simulink model "Pilote_SimMechanics"  (R2013a)
settings: Solver=ode15s  StartTime=0.0  StopTime=10.0  RelTol=1e-3
undefined symbols (not defined in the file): _EF_BancPH_ivan, RootGround, RootPart, SE_Bati, SE_Cylindre, SE_Safran
libraries: mblibv1 x14
settings Model: Creator=Ivan  LastModifiedBy=Ivan
settings SimMechanicsCC: VisOnUpdateDiagram=on  VisDuringSimulation=on

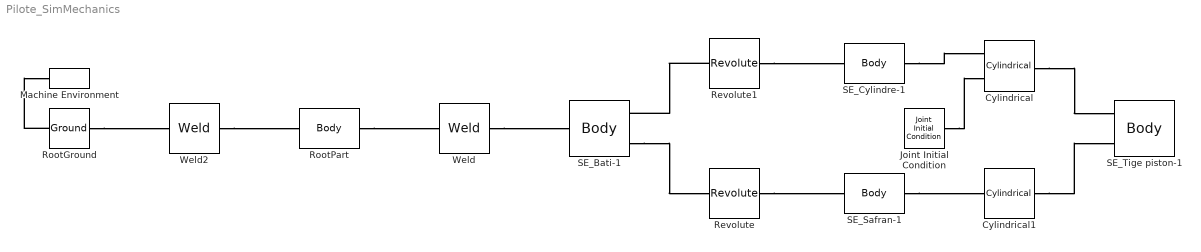
== system Pilote_SimMechanics ==
  Cylindrical : mblibv1/Joints/Cylindrical  LConnTagsString=__newl0|SA1  RConnTagsString=__newr0  UpdateFromCAD=on  PMImportedID=SE_Cylindre-1:-:SE_Tige piston-1  NumSAPorts=1  CutJoint=off  MarkAsCut=off  Primitives=prismatic  PrimitiveProps=P1$World$[-0.999105,-0.0423027,0]$prismatic#R1$World$[-0.999105,-0.0423027,0]$revolute  DialogClass=JointBlock  P1Axis=[-0.999105,-0.0423027,0]  R1Axis=[-0.999105,-0.0423027,0]
  Cylindrical1 : mblibv1/Joints/Cylindrical  LConnTagsString=__newl0  RConnTagsString=__newr0  UpdateFromCAD=on  PMImportedID=SE_Safran-1:-:SE_Tige piston-1  NumSAPorts=0  CutJoint=off  MarkAsCut=off  Primitives=prismatic  PrimitiveProps=P1$WORLD$[0,0,-1]$prismatic#R1$WORLD$[0,0,-1]$revolute  DialogClass=JointBlock  P1Axis=[0,0,-1]  R1Axis=[0,0,-1]
  Joint Initial Condition : mblibv1/Sensors &  Actuators/Joint Initial Condition  UpdateFromCAD=off  LeftPortType=blob  RightPortType=blob  PhysicalDomain=mechanical  DialogClass=InitialConditionBlock  InitialConditions=P1$true$0$m$deg$1$cm/s$deg/s#P2$false$0$m$deg$0$m/s$deg/s#P3$false$0$m$deg$0$m/s$deg/s#R1$false$0$m$deg$0$m/s$deg/s#R2$false$0$m$deg$0$m/s$deg/s#R3$false$0$m$deg$0$m/s$deg/s#S$false$0$m$deg$0$m/s$deg/s  P1PIC=0  P1VIC=1  P2PIC=0  P2VIC=0  P3PIC=0  P3VIC=0  R1PIC=0  R1VIC=0  R2PIC=0  R2VIC=0  R3PIC=0  R3VIC=0  SPIC=0  SVIC=0
  Machine Environment : mblibv1/Bodies/Machine Environment  PortType=env  PhysicalDomain=Mechanical  DialogTemplateClass=MECH.MachineEnvironment  SyncWhenCopied=off  Gravity=[0 0 -9.81]  GravityUnits=m/s^2  GravityAsSignal=off  Dimensionality=Auto-detect  AnalysisType=Forward dynamics  LinearAssemblyTolerance=1e-3  LinearAssemblyToleranceUnits=m  AngularAssemblyTolerance=1e-3  AngularAssemblyToleranceUnits=rad  ConstraintSolverType=Stabilizing  ConstraintRelTolerance=1e-4  ConstraintAbsTolerance=1e-4  UseRobustSingularityHandling=off  RedundancyAnalysisToleranceType=Automatically select tolerance  RedundancyAnalysisTolerance=1e-14  StatePerturbationType=Fixed  PerturbationSize=1e-5  VisualizeMachine=on  BodyVisualizationType=Use model default body geometries  BodyColorSelMode=Use model default  DefaultBodyColor=[1 0 0]
  Revolute : mblibv1/Joints/Revolute  LConnTagsString=__newl0  RConnTagsString=__newr0  UpdateFromCAD=on  PMImportedID=SE_Bati-1:-:SE_Safran-1  NumSAPorts=0  CutJoint=off  MarkAsCut=off  Primitives=prismatic  PrimitiveProps=R1$WORLD$[0,0,1]$revolute  DialogClass=JointBlock  R1Axis=[0,0,1]
  Revolute1 : mblibv1/Joints/Revolute  LConnTagsString=__newl0  RConnTagsString=__newr0  UpdateFromCAD=off  NumSAPorts=0  CutJoint=off  MarkAsCut=off  Primitives=prismatic  PrimitiveProps=R1$World$[0 0 1]$revolute  DialogClass=JointBlock  R1Axis=[0 0 1]
  RootGround : mblibv1/Bodies/Ground  UpdateFromCAD=on  PMImportedID=RootGround  LeftPortType=env  RightPortType=workingframe  PhysicalDomain=Mechanical  DialogClass=GroundBlock  CoordPosition=[-1.08828,0.614921,0.309081]  CoordPositionUnits=m  StateVectorMgrId=0  MachineId=[1 0]  ShowEnvPort=on
  RootPart : mblibv1/Bodies/Body  LConnTagsString=CS3  RConnTagsString=CS2  UpdateFromCAD=on  PMImportedID=_EF_BancPH_ivan/RootPart  DialogClass=MechanicalBodyBlock  Mass=0  MassUnits=kg  InertiaUnits=kg*m^2  Inertia=[0,0,0;0,0,0;0,0,0]  Shape=Cylinder  ShapeDims=[1 1]  ShapeUnits=m  ShapeUse=false  Density=1  DensityUnits=kg/m^3  DensityUse=false  GraphicsMode=MACHINE_DEFAULT  BodyColorSelMode=MACHINE_DEFAULT  BodyColor=[1;0;0]  AttachedToCS=CS1  CG=Right$CG$[-1.08828 0.614921 0.309081]$WORLD$WORLD$m$[1 0 0;0 1 0;0 0 1]$3x3 Transform$rad$WORLD$false$_EF_BancPH_ivan/RootPart::CG(AUTOGEN)  WorkingFrames=Right$CS1$[0 0 0]$WORLD$WORLD$m$[1 0 0;0 1 0;0 0 1]$3x3 Transform$rad$WORLD$false$_EF_BancPH_ivan/RootPart::CS1(AUTOGEN)#Right$CS2$[-1.08627 0.612468 0.301696]$WORLD$WORLD$m$[1 0 0;0 1 0;0 0 1]$3x3 Transform$rad$WORLD$true$SE_Bati-1:-:_EF_BancPH_ivan/RootPart::_EF_BancPH_ivan/RootPart(AUTOGEN)#Left$CS3$[-1.08828 0.614921 0.309081]$WORLD$WORLD$m$[1 0 0;0 1 0;0 0 1]$3x3 Transform$rad$WORLD$true$RootGround:-:_EF_BancPH_ivan/RootPart::_EF_BancPH_ivan/RootPart(AUTOGEN)  CGPos=[-1.08828 0.614921 0.309081]  CGRot=[1 0 0;0 1 0;0 0 1]  CS0Pos=[]  CS0Rot=[]  CS1Pos=[0 0 0]  CS1Rot=[1 0 0;0 1 0;0 0 1]  CS2Pos=[-1.08627 0.612468 0.301696]  CS2Rot=[1 0 0;0 1 0;0 0 1]  CS3Pos=[-1.08828 0.614921 0.309081]  CS3Rot=[1 0 0;0 1 0;0 0 1]  CS4Pos=[]  CS4Rot=[]  CS5Pos=[]  CS5Rot=[]  CS6Pos=[]  CS6Rot=[]  CS7Pos=[]  CS7Rot=[]  CS8Pos=[]  CS8Rot=[]  CS9Pos=[]  CS9Rot=[]  CS10Pos=[]  CS10Rot=[]  CS11Pos=[]  CS11Rot=[]  CS12Pos=[]  CS12Rot=[]  CS13Pos=[]  CS13Rot=[]  CS14Pos=[]  CS14Rot=[]  CS15Pos=[]  CS15Rot=[]  CS16Pos=[]  CS16Rot=[]  CS17Pos=[]  CS17Rot=[]  CS18Pos=[]  CS18Rot=[]  CS19Pos=[]  CS19Rot=[]  CS20Pos=[]  CS20Rot=[]
  SE_Bati-1 : mblibv1/Bodies/Body  LConnTagsString=CS2  RConnTagsString=CS3|CS4  UpdateFromCAD=on  PMImportedID=SE_Bati-1  DialogClass=MechanicalBodyBlock  Mass=10.7703  MassUnits=kg  InertiaUnits=kg*m^2  Inertia=[0.196607,0.0119133,0.0109935;0.0119133,1.14271,-0.000206125;0.0109935,-0.000206125,1.29701]  Shape=Cylinder  ShapeDims=[1 1]  ShapeUnits=m  ShapeUse=false  Density=1  DensityUnits=kg/m^3  DensityUse=false  GraphicsMode=GFXFILE  GraphicsFileName=_EF_BancPH_ivan - SE_Bati-1.STL  BodyColorSelMode=COLORPALETTE  BodyColor=[0.752941;0.752941;0.752941]  AttachedToCS=CS1  CG=Right$CG$[-1.08627 0.612468 0.301696]$WORLD$WORLD$m$[1 0 0;0 1 0;0 0 1]$3x3 Transform$rad$WORLD$false$SE_Bati-1::CG(AUTOGEN)  WorkingFrames=Right$CS1$[-0.854297 0.517993 0.336389]$WORLD$WORLD$m$[1 0 0;0 1 0;0 0 1]$3x3 Transform$rad$WORLD$false$SE_Bati-1::CS1(AUTOGEN)#Left$CS2$[-1.08627 0.612468 0.301696]$WORLD$WORLD$m$[1 0 0;0 1 0;0 0 1]$3x3 Transform$rad$WORLD$true$SE_Bati-1:-:_EF_BancPH_ivan/RootPart::SE_Bati-1(AUTOGEN)#Right$CS3$[-1.4478 0.672993 0.391315]$WORLD$WORLD$m$[1 0 0;0 1 0;0 0 1]$3x3 Transform$rad$WORLD$true$SE_Bati-1:-:SE_Cylindre-1::SE_Bati-1(AUTOGEN)#Right$CS4$[-0.854297 0.517993 0.340389]$WORLD$WORLD$m$[1 0 0;0 1 0;0 0 1]$3x3 Transform$rad$WORLD$true$SE_Bati-1:-:SE_Safran-1::SE_Bati-1(AUTOGEN)  CGPos=[-1.08627 0.612468 0.301696]  CGRot=[1 0 0;0 1 0;0 0 1]  CS0Pos=[]  CS0Rot=[]  CS1Pos=[-0.854297 0.517993 0.336389]  CS1Rot=[1 0 0;0 1 0;0 0 1]  CS2Pos=[-1.08627 0.612468 0.301696]  CS2Rot=[1 0 0;0 1 0;0 0 1]  CS3Pos=[-1.4478 0.672993 0.391315]  CS3Rot=[1 0 0;0 1 0;0 0 1]  CS4Pos=[-0.854297 0.517993 0.340389]  CS4Rot=[1 0 0;0 1 0;0 0 1]  CS5Pos=[]  CS5Rot=[]  CS6Pos=[]  CS6Rot=[]  CS7Pos=[]  CS7Rot=[]  CS8Pos=[]  CS8Rot=[]  CS9Pos=[]  CS9Rot=[]  CS10Pos=[]  CS10Rot=[]  CS11Pos=[]  CS11Rot=[]  CS12Pos=[]  CS12Rot=[]  CS13Pos=[]  CS13Rot=[]  CS14Pos=[]  CS14Rot=[]  CS15Pos=[]  CS15Rot=[]  CS16Pos=[]  CS16Rot=[]  CS17Pos=[]  CS17Rot=[]  CS18Pos=[]  CS18Rot=[]  CS19Pos=[]  CS19Rot=[]  CS20Pos=[]  CS20Rot=[]
  SE_Cylindre-1 : mblibv1/Bodies/Body  LConnTagsString=CS3  RConnTagsString=CS2  UpdateFromCAD=on  PMImportedID=SE_Cylindre-1  DialogClass=MechanicalBodyBlock  Mass=0.415934  MassUnits=kg  InertiaUnits=kg*m^2  Inertia=[0.000227172,1.52435e-05,-8.18122e-06;1.52435e-05,0.00749454,-2.83709e-06;-8.18122e-06,-2.83709e-06,0.00748907]  Shape=Cylinder  ShapeDims=[1 1]  ShapeUnits=m  ShapeUse=false  Density=1  DensityUnits=kg/m^3  DensityUse=false  GraphicsMode=GFXFILE  GraphicsFileName=_EF_BancPH_ivan - SE_Cylindre-1.STL  BodyColorSelMode=COLORPALETTE  BodyColor=[0.305882;0.305882;0.305882]  AttachedToCS=CS1  CG=Right$CG$[-1.24889 0.681158 0.405388]$WORLD$WORLD$m$[0.999105 -0.0372355 0.0200757;0.0423027 0.879429 -0.474147;0 0.474572 0.880217]$3x3 Transform$rad$WORLD$false$SE_Cylindre-1::CG(AUTOGEN)  WorkingFrames=Right$CS1$[-1.2867 0.567246 0.418732]$WORLD$WORLD$m$[0.999105 -0.0372355 0.0200757;0.0423027 0.879429 -0.474147;0 0.474572 0.880217]$3x3 Transform$rad$WORLD$false$SE_Cylindre-1::CS1(AUTOGEN)#Right$CS2$[-1.10291 0.687596 0.405389]$WORLD$WORLD$m$[1 0 0;0 1 0;0 0 1]$3x3 Transform$rad$WORLD$true$SE_Cylindre-1:-:SE_Tige piston-1::SE_Cylindre-1(AUTOGEN)#Left$CS3$[-1.4478 0.672993 0.391315]$WORLD$WORLD$m$[1 0 0;0 1 0;0 0 1]$3x3 Transform$rad$WORLD$true$SE_Bati-1:-:SE_Cylindre-1::SE_Cylindre-1(AUTOGEN)  CGPos=[-1.24889 0.681158 0.405388]  CGRot=[0.999105 -0.0372355 0.0200757;0.0423027 0.879429 -0.474147;0 0.474572 0.880217]  CS0Pos=[]  CS0Rot=[]  CS1Pos=[-1.2867 0.567246 0.418732]  CS1Rot=[0.999105 -0.0372355 0.0200757;0.0423027 0.879429 -0.474147;0 0.474572 0.880217]  CS2Pos=[-1.10291 0.687596 0.405389]  CS2Rot=[1 0 0;0 1 0;0 0 1]  CS3Pos=[-1.4478 0.672993 0.391315]  CS3Rot=[1 0 0;0 1 0;0 0 1]  CS4Pos=[]  CS4Rot=[]  CS5Pos=[]  CS5Rot=[]  CS6Pos=[]  CS6Rot=[]  CS7Pos=[]  CS7Rot=[]  CS8Pos=[]  CS8Rot=[]  CS9Pos=[]  CS9Rot=[]  CS10Pos=[]  CS10Rot=[]  CS11Pos=[]  CS11Rot=[]  CS12Pos=[]  CS12Rot=[]  CS13Pos=[]  CS13Rot=[]  CS14Pos=[]  CS14Rot=[]  CS15Pos=[]  CS15Rot=[]  CS16Pos=[]  CS16Rot=[]  CS17Pos=[]  CS17Rot=[]  CS18Pos=[]  CS18Rot=[]  CS19Pos=[]  CS19Rot=[]  CS20Pos=[]  CS20Rot=[]
  SE_Safran-1 : mblibv1/Bodies/Body  LConnTagsString=CS3  RConnTagsString=CS2  UpdateFromCAD=on  PMImportedID=SE_Safran-1  DialogClass=MechanicalBodyBlock  Mass=0.316611  MassUnits=kg  InertiaUnits=kg*m^2  Inertia=[0.000714938,6.94962e-06,-0.000382637;6.94962e-06,0.00187569,-1.56573e-06;-0.000382637,-1.56573e-06,0.00126027]  Shape=Cylinder  ShapeDims=[1 1]  ShapeUnits=m  ShapeUse=false  Density=1  DensityUnits=kg/m^3  DensityUse=false  GraphicsMode=GFXFILE  GraphicsFileName=_EF_BancPH_ivan - SE_Safran-1.STL  BodyColorSelMode=COLORPALETTE  BodyColor=[0.752941;0.752941;0.752941]  AttachedToCS=CS1  CG=Right$CG$[-0.855465 0.553018 0.352112]$WORLD$WORLD$m$[-0.0234219 -0.999726 0;0.999726 -0.0234219 0;0 0 1]$3x3 Transform$rad$WORLD$false$SE_Safran-1::CG(AUTOGEN)  WorkingFrames=Right$CS1$[-0.854297 0.517993 0.393889]$WORLD$WORLD$m$[-0.0234219 -0.999726 0;0.999726 -0.0234219 0;0 0 1]$3x3 Transform$rad$WORLD$false$SE_Safran-1::CS1(AUTOGEN)#Right$CS2$[-0.858513 0.697944 0.420889]$WORLD$WORLD$m$[1 0 0;0 1 0;0 0 1]$3x3 Transform$rad$WORLD$true$SE_Safran-1:-:SE_Tige piston-1::SE_Safran-1(AUTOGEN)#Left$CS3$[-0.854297 0.517993 0.340389]$WORLD$WORLD$m$[1 0 0;0 1 0;0 0 1]$3x3 Transform$rad$WORLD$true$SE_Bati-1:-:SE_Safran-1::SE_Safran-1(AUTOGEN)  CGPos=[-0.855465 0.553018 0.352112]  CGRot=[-0.0234219 -0.999726 0;0.999726 -0.0234219 0;0 0 1]  CS0Pos=[]  CS0Rot=[]  CS1Pos=[-0.854297 0.517993 0.393889]  CS1Rot=[-0.0234219 -0.999726 0;0.999726 -0.0234219 0;0 0 1]  CS2Pos=[-0.858513 0.697944 0.420889]  CS2Rot=[1 0 0;0 1 0;0 0 1]  CS3Pos=[-0.854297 0.517993 0.340389]  CS3Rot=[1 0 0;0 1 0;0 0 1]  CS4Pos=[]  CS4Rot=[]  CS5Pos=[]  CS5Rot=[]  CS6Pos=[]  CS6Rot=[]  CS7Pos=[]  CS7Rot=[]  CS8Pos=[]  CS8Rot=[]  CS9Pos=[]  CS9Rot=[]  CS10Pos=[]  CS10Rot=[]  CS11Pos=[]  CS11Rot=[]  CS12Pos=[]  CS12Rot=[]  CS13Pos=[]  CS13Rot=[]  CS14Pos=[]  CS14Rot=[]  CS15Pos=[]  CS15Rot=[]  CS16Pos=[]  CS16Rot=[]  CS17Pos=[]  CS17Rot=[]  CS18Pos=[]  CS18Rot=[]  CS19Pos=[]  CS19Rot=[]  CS20Pos=[]  CS20Rot=[]
  SE_Tige piston-1 : mblibv1/Bodies/Body  LConnTagsString=CS2|CS3  UpdateFromCAD=on  PMImportedID=SE_Tige piston-1  DialogClass=MechanicalBodyBlock  Mass=0.268512  MassUnits=kg  InertiaUnits=kg*m^2  Inertia=[2.06372e-05,3.05648e-08,6.48832e-11;3.05648e-08,0.012085,-8.15232e-11;6.48832e-11,-8.15232e-11,0.0120871]  Shape=Cylinder  ShapeDims=[1 1]  ShapeUnits=m  ShapeUse=false  Density=1  DensityUnits=kg/m^3  DensityUse=false  GraphicsMode=GFXFILE  GraphicsFileName=_EF_BancPH_ivan - SE_Tige piston-1.STL  BodyColorSelMode=COLORPALETTE  BodyColor=[0.752941;0.752941;0.752941]  AttachedToCS=CS1  CG=Right$CG$[-1.19461 0.683713 0.405389]$WORLD$WORLD$m$[0.999105 0.0423027 0;0.0423027 -0.999105 0;0 0 -1]$3x3 Transform$rad$WORLD$false$SE_Tige piston-1::CG(AUTOGEN)  WorkingFrames=Right$CS1$[-1.43849 0.673387 0.405389]$WORLD$WORLD$m$[0.999105 0.0423027 0;0.0423027 -0.999105 0;0 0 -1]$3x3 Transform$rad$WORLD$false$SE_Tige piston-1::CS1(AUTOGEN)#Left$CS2$[-1.10291 0.687596 0.405389]$WORLD$WORLD$m$[1 0 0;0 1 0;0 0 1]$3x3 Transform$rad$WORLD$true$SE_Cylindre-1:-:SE_Tige piston-1::SE_Tige piston-1(AUTOGEN)#Left$CS3$[-0.858513 0.697944 0.420889]$WORLD$WORLD$m$[1 0 0;0 1 0;0 0 1]$3x3 Transform$rad$WORLD$true$SE_Safran-1:-:SE_Tige piston-1::SE_Tige piston-1(AUTOGEN)  CGPos=[-1.19461 0.683713 0.405389]  CGRot=[0.999105 0.0423027 0;0.0423027 -0.999105 0;0 0 -1]  CS0Pos=[]  CS0Rot=[]  CS1Pos=[-1.43849 0.673387 0.405389]  CS1Rot=[0.999105 0.0423027 0;0.0423027 -0.999105 0;0 0 -1]  CS2Pos=[-1.10291 0.687596 0.405389]  CS2Rot=[1 0 0;0 1 0;0 0 1]  CS3Pos=[-0.858513 0.697944 0.420889]  CS3Rot=[1 0 0;0 1 0;0 0 1]  CS4Pos=[]  CS4Rot=[]  CS5Pos=[]  CS5Rot=[]  CS6Pos=[]  CS6Rot=[]  CS7Pos=[]  CS7Rot=[]  CS8Pos=[]  CS8Rot=[]  CS9Pos=[]  CS9Rot=[]  CS10Pos=[]  CS10Rot=[]  CS11Pos=[]  CS11Rot=[]  CS12Pos=[]  CS12Rot=[]  CS13Pos=[]  CS13Rot=[]  CS14Pos=[]  CS14Rot=[]  CS15Pos=[]  CS15Rot=[]  CS16Pos=[]  CS16Rot=[]  CS17Pos=[]  CS17Rot=[]  CS18Pos=[]  CS18Rot=[]  CS19Pos=[]  CS19Rot=[]  CS20Pos=[]  CS20Rot=[]
  Weld : mblibv1/Joints/Weld  LConnTagsString=__newl0  RConnTagsString=__newr0  UpdateFromCAD=on  PMImportedID=SE_Bati-1:-:_EF_BancPH_ivan/RootPart  NumSAPorts=0  CutJoint=off  MarkAsCut=off  Primitives=weld  PrimitiveProps=W$WORLD$[0.57735,0.57735,0.57735]$weld  DialogClass=JointBlock  WAxis=[0.57735,0.57735,0.57735]
  Weld2 : mblibv1/Joints/Weld  LConnTagsString=__newl0  RConnTagsString=__newr0  UpdateFromCAD=on  PMImportedID=RootGround:-:_EF_BancPH_ivan/RootPart  NumSAPorts=0  CutJoint=off  MarkAsCut=off  Primitives=weld  PrimitiveProps=W$WORLD$[0.57735,0.57735,0.57735]$weld  DialogClass=JointBlock  WAxis=[0.57735,0.57735,0.57735]
  connections:
  RootPart/RConn1 -- Weld/LConn1
  Weld/RConn1 -- SE_Bati-1/LConn1
  SE_Safran-1/RConn1 -- Cylindrical1/LConn1
  Cylindrical1/RConn1 -- SE_Tige piston-1/LConn2
  Revolute1/LConn1 -- SE_Bati-1/RConn1
  Revolute1/RConn1 -- SE_Cylindre-1/LConn1
  SE_Bati-1/RConn2 -- Revolute/LConn1
  Revolute/RConn1 -- SE_Safran-1/LConn1
  RootGround/RConn1 -- Weld2/LConn1
  Weld2/RConn1 -- RootPart/LConn1
  RootGround/LConn1 -- Machine Environment/RConn1
  SE_Cylindre-1/RConn1 -- Cylindrical/LConn1
  Cylindrical/RConn1 -- SE_Tige piston-1/LConn1
  Joint Initial Condition/RConn1 -- Cylindrical/LConn2
